simulink model "msap_new"  (R2019b)
settings: Solver=VariableStepAuto  StartTime=0.0  StopTime=2  RelTol=1e-3
InitFcn:
  | % Paramètres (Test initial)
  | clc;
  | clear all;
  | 
  | Rs = 0.8;        % Résistance statorique
  | Ld = 1.10e-3;     % Inductance axe d
  | Lq = 1.32e-3;     % Inductance axe q
  | %Qf=1.5;        % Flux des aimants (Phi_f)
  | p = 2;           % Nombre de paires de pôles
  | J = 1.15e-3;     % Moment d'inertie
  | fr = 0.59e-2;     % Coefficient de frottement
  | 
  | 
  | 
  | 
  | 
  | 
  | Qf= 0.12;       % Flux des aimants (Phi_f)
libraries: simulink x1
settings Model: Creator=x1 yoga  LastModifiedBy=x1 yoga

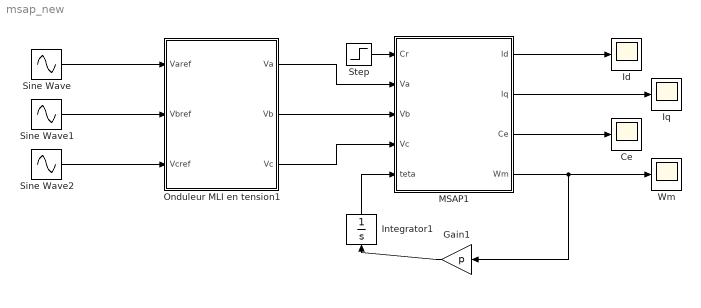
== system msap_new ==
  " MSAP1" : Subsystem
  Ce : Scope
  Gain1 : Gain  Gain=p
  Id : Scope
  Integrator1 : Integrator
  Iq : Scope
  Onduleur MLI en tension1 : Subsystem
  Sine Wave : Sin  Amplitude=100  Frequency=2*pi*50  SampleTime=0
  Sine Wave1 : Sin  Amplitude=100  Frequency=2*pi*50  Phase=-2*pi/3  SampleTime=0
  Sine Wave2 : Sin  Amplitude=100  Frequency=2*pi*50  Phase=2*pi/3  SampleTime=0
  Step : Step  After=5  SampleTime=0
  Wm : Scope
  wires:
  Gain1/1 -> Integrator1/1
  " MSAP1"/3(Ce) -> Ce/1
  " MSAP1"/1(Id) -> Id/1
  Step/1 -> " MSAP1"/1(Cr)
  Onduleur MLI en tension1/2(Vb) -> " MSAP1"/3(Vb)
  Sine Wave2/1 -> Onduleur MLI en tension1/3(Vcref)
  Onduleur MLI en tension1/3(Vc) -> " MSAP1"/4(Vc)
  " MSAP1"/2(Iq) -> Iq/1
  Onduleur MLI en tension1/1(Va) -> " MSAP1"/2(Va)
  " MSAP1"/4("Wm ") -> Gain1/1, Wm/1
  Sine Wave/1 -> Onduleur MLI en tension1/1(Varef)
  Integrator1/1 -> " MSAP1"/5(teta)
  Sine Wave1/1 -> Onduleur MLI en tension1/2(Vbref)

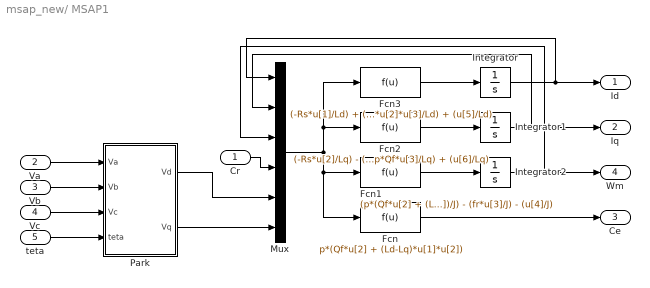
== system msap_new/ MSAP1 ==
  Cr : Inport
  Va : Inport  Port=2
  Vb : Inport  Port=3
  Vc : Inport  Port=4
  teta : Inport  Port=5
  Fcn : Fcn  Expr=p*(Qf*u[2] + (Ld-Lq)*u[1]*u[2])
  Fcn1 : Fcn  Expr=(p*(Qf*u[2] + (Ld-Lq)*u[1]*u[2])/J) - (fr*u[3]/J) - (u[4]/J)
  Fcn2 : Fcn  Expr=(-Rs*u[2]/Lq) - (p*Ld*u[3]*u[1]/Lq) - (p*Qf*u[3]/Lq) + (u[6]/Lq)
  Fcn3 : Fcn  Expr=(-Rs*u[1]/Ld) + (p*Lq*u[2]*u[3]/Ld) + (u[5]/Ld)
  Integrator : Integrator
  Integrator1 : Integrator
  Integrator2 : Integrator
  Mux : Mux  Inputs=6
  Park : Subsystem
  Id : Outport
  Iq : Outport  Port=2
  Ce : Outport  Port=3
  "Wm " : Outport  Port=4
  wires:
  Mux/1 -> Fcn1/1, Fcn/1, Fcn2/1, Fcn3/1
  Fcn/1 -> Ce/1
  Integrator1/1 -> Iq/1, Mux/2
  Vb/1 -> Park/2(Vb)
  Integrator2/1 -> "Wm "/1, Mux/3
  Integrator/1 -> Id/1, Mux/1
  Fcn2/1 -> Integrator1/1
  Park/2("Vq ") -> Mux/6
  Cr/1 -> Mux/4
  Park/1("Vd ") -> Mux/5
  Va/1 -> Park/1(Va)
  Vc/1 -> Park/3(Vc)
  Fcn3/1 -> Integrator/1
  teta/1 -> Park/4(teta)
  Fcn1/1 -> Integrator2/1

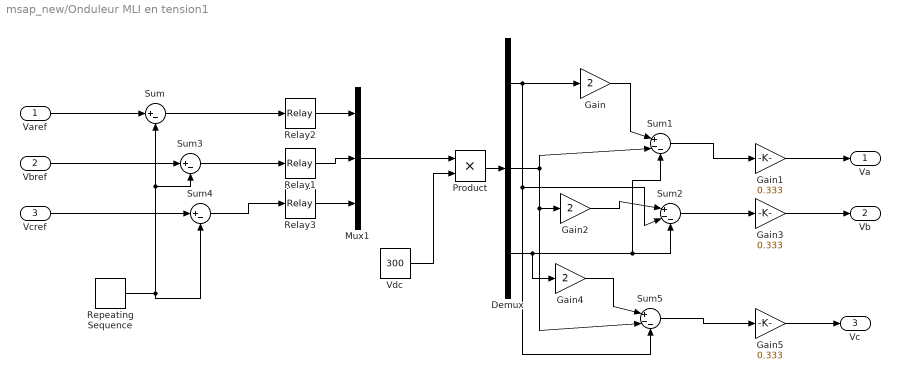
== system msap_new/Onduleur MLI en tension1 ==
  Varef : Inport
  Vbref : Inport  Port=2
  Vcref : Inport  Port=3
  Demux : Demux  Outputs=3
  Gain : Gain  Gain=2
  Gain1 : Gain  Gain=0.333
  Gain2 : Gain  Gain=2
  Gain3 : Gain  Gain=0.333
  Gain4 : Gain  Gain=2
  Gain5 : Gain  Gain=0.333
  Mux1 : Mux  Inputs=3
  Product : Product
  Relay1 : Relay
  Relay2 : Relay
  Relay3 : Relay
  Repeating Sequence : simulink/Sources/Repeating Sequence  rep_seq_t=[0 0.00025 0.0005]  rep_seq_y=[0 1 0]
  Sum : Sum  Inputs=|+-
  Sum1 : Sum  Inputs=|+--
  Sum2 : Sum  Inputs=|+--
  Sum3 : Sum  Inputs=|+-
  Sum4 : Sum  Inputs=|+-
  Sum5 : Sum  Inputs=|+--
  "Vdc " : Constant  Value=300
  Va : Outport
  Vb : Outport  Port=2
  Vc : Outport  Port=3
  wires:
  "Vdc "/1 -> Product/2
  Relay3/1 -> Mux1/3
  Gain4/1 -> Sum5/1
  Repeating Sequence/1 -> Sum4/2, Sum3/2, Sum/2
  Demux/1 -> Sum5/3, Sum2/2, Gain/1
  Demux/3 -> Gain4/1, Sum2/3, Sum1/3
  Sum4/1 -> Relay3/1
  Demux/2 -> Sum5/2, Gain2/1, Sum1/2
  Varef/1 -> Sum/1
  Gain2/1 -> Sum2/1
  Sum/1 -> Relay2/1
  Relay2/1 -> Mux1/1
  Sum1/1 -> Gain1/1
  Product/1 -> Demux/1
  Vcref/1 -> Sum4/1
  Sum2/1 -> Gain3/1
  Sum3/1 -> Relay1/1
  Vbref/1 -> Sum3/1
  Relay1/1 -> Mux1/2
  Sum5/1 -> Gain5/1
  Mux1/1 -> Product/1
  Gain/1 -> Sum1/1
  Gain5/1 -> Vc/1
  Gain3/1 -> Vb/1
  Gain1/1 -> Va/1

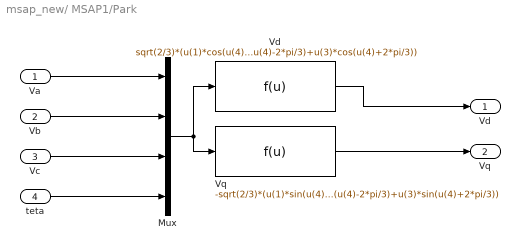
== system msap_new/ MSAP1/Park ==
  Va : Inport
  Vb : Inport  Port=2
  Vc : Inport  Port=3
  teta : Inport  Port=4
  Mux : Mux
  Vd : Fcn  Expr=sqrt(2/3)*(u(1)*cos(u(4))+u(2)*cos(u(4)-2*pi/3)+u(3)*cos(u(4)+2*pi/3))
  Vq : Fcn  Expr=-sqrt(2/3)*(u(1)*sin(u(4))+u(2)*sin(u(4)-2*pi/3)+u(3)*sin(u(4)+2*pi/3))
  "Vd " : Outport
  "Vq " : Outport  Port=2
  wires:
  Vq/1 -> "Vq "/1
  Vd/1 -> "Vd "/1
  Vb/1 -> Mux/2
  Mux/1 -> Vq/1, Vd/1
  Va/1 -> Mux/1
  Vc/1 -> Mux/3
  teta/1 -> Mux/4
